simulink model "MMS_ESC_K_B_dither_free"  (R2019b)
settings: Solver=ode4  StartTime=par.sym.TStart  StopTime=par.sym.TStop  FixedStep=par.sym.max_dt  MaxStep=par.sym.max_dt  RelTol=1e-3
undefined symbols (not defined in the file): a1, a1_B, amp, amp_B, b, B_0, B_init, k, K_0, k_B, K_init, k_K, m, N_buff_B, N_buff_K, N_delay, omega, par, R, R_B, T_tran, w_L_B, w_L_K, w_wav
libraries: simulink x2
settings Model: Creator=Vitù  LastModifiedBy=User
settings DataIOCC: SaveFormat=Array  SaveOutput=off  SignalLogging=off  DSMLogging=off  ReturnWorkspaceOutputs=off  TimeSaveName=TIME  OutputSaveName=Yout  OutputOption=SpecifiedOutputTimes  OutputTimes=[par.sym.TStart:par.sym.Outputdt:par.sym.TStop]
settings OptimizationCC: ExpressionDepthLimit=2147483647  LifeSpan=inf
settings DebuggingCC: UnderspecifiedInitializationDetection=Classic  MergeDetectMultiDrivingBlocksExec=none  SolverPrmCheckMsg=warning  AllowSymbolicDim=off  StateNameClashWarn=warning  SFUnexpectedBacktrackingDiag=warning  SFNoUnconditionalDefaultTransitionDiag=warning  SFExecutionAtInitializationDiag=none  ArithmeticOperatorsInVariantConditions=warning
settings HardwareCC: ProdBitPerPointer=32  ProdBitPerSizeT=32  ProdBitPerPtrDiffT=32  ProdLargestAtomicFloat=None  ProdIntDivRoundTo=Undefined  ProdEndianess=Unspecified  ProdWordSize=32  ProdHWDeviceType=32-bit Generic
settings ModelReferenceCC: PropagateSignalLabelsOutOfModel=off
settings SFSimCC: SimUseLocalCustomCode=off  CustomCodeUndefinedFunction=UseInterfaceOnly
settings RTWCC: RTWUseLocalCustomCode=off
settings CodeAppCC: StateflowObjectComments=on
settings GRTTargetCC: TargetLangStandard=C89/C90 (ANSI)  GeneratePreprocessorConditionals=Disable all
settings ConfigComp: CovMetricSettings=dw  CovHtmlReporting=on  CovSaveCumulativeToWorkspaceVar=on  CovSaveSingleToWorkspaceVar=on  CovExternalEMLEnable=off  CovSFcnEnable=off
settings SimscapeCC: SimscapeNormalizeSystem=off
settings ConfigurationSet: Description=SimMechanics 2G

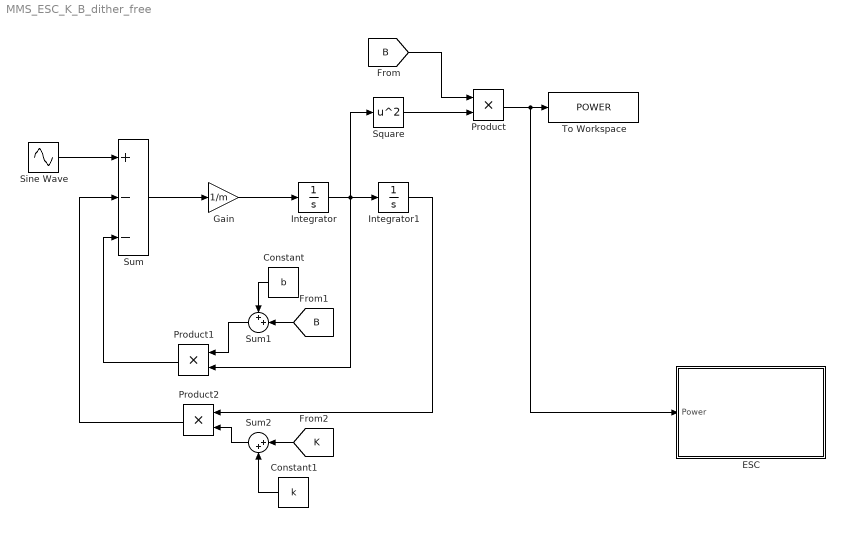
== system MMS_ESC_K_B_dither_free ==
  Constant : Constant  Value=b
  Constant1 : Constant  Value=k
  ESC : Subsystem
  Gain : Gain  Gain=1/m
  Integrator : Integrator
  Integrator1 : Integrator
  Product : Product
  Product1 : Product
  Product2 : Product
  Sine Wave : Sin  Amplitude=par.H  Frequency=w_wav  SampleTime=0
  Square : Math  Operator=square  SignedPower=off  SaturateOnIntegerOverflow=on
  Sum : Sum  Inputs=+--
  Sum1 : Sum  Inputs=++|
  Sum2 : Sum  Inputs=|++
  To Workspace : ToWorkspace  VariableName=POWER  SampleTime=-1
  wires:
  Integrator1/1 -> Product2/1
  Product/1 -> ESC/1(Power), To Workspace/1
  Product1/1 -> Sum/3
  Gain/1 -> Integrator/1
  Square/1 -> Product/2
  Sum/1 -> Gain/1
  Integrator/1 -> Product1/2, Square/1, Integrator1/1
  Product2/1 -> Sum/2
  Sine Wave/1 -> Sum/1
  [B] -> Product/1
  [B] -> Sum1/2
  Sum1/1 -> Product1/1
  Constant/1 -> Sum1/1
  [K] -> Sum2/1
  Sum2/1 -> Product2/2
  Constant1/1 -> Sum2/2

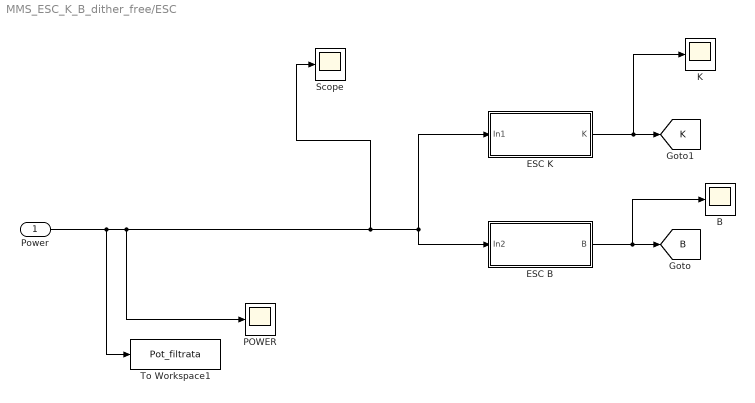
== system MMS_ESC_K_B_dither_free/ESC ==
  Power : Inport
  B : Scope
  ESC B : Subsystem
  ESC K : Subsystem
  K : Scope
  POWER : Scope
  Scope : Scope
  To Workspace1 : ToWorkspace  VariableName=Pot_filtrata  SampleTime=-1
  tag scope: B=global, K=global
  wires:
  Power/1 -> ESC B/1(In2), ESC K/1(In1), Scope/1, POWER/1, To Workspace1/1
  ESC B/1(B) -> B/1, [B]
  ESC K/1(K) -> K/1, [K]

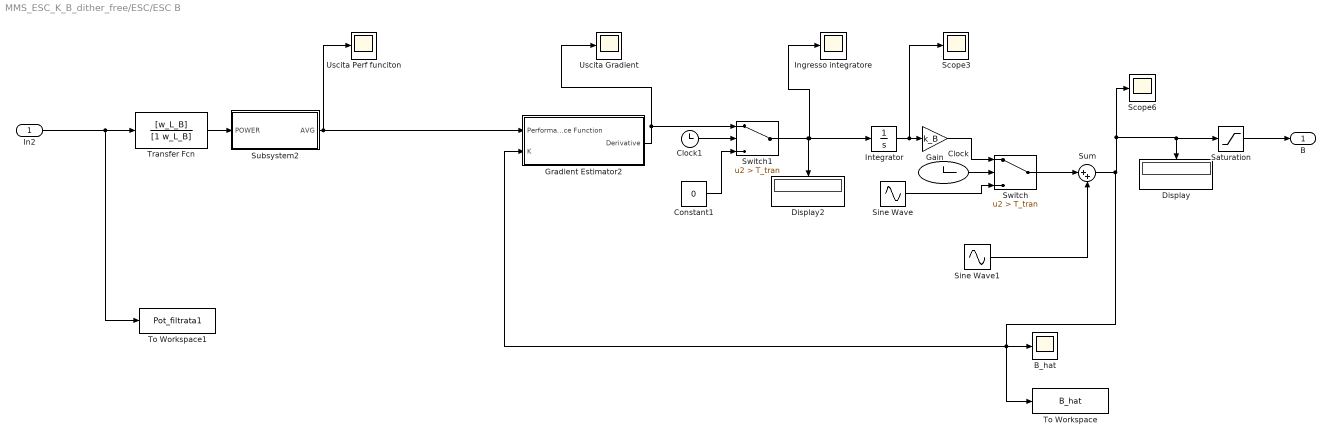
== system MMS_ESC_K_B_dither_free/ESC/ESC B ==
  In2 : Inport
  B_hat : Scope
  Clock : Clock
  Clock1 : Clock
  Constant1 : Constant  Value=0
  Display : Display
  Display2 : Display
  Gain : Gain  Gain=k_B
  Gradient Estimator2 : Subsystem
  Ingresso integratore : Scope
  Integrator : Integrator  InitialCondition=B_init
  Saturation : Saturate  UpperLimit=inf  LowerLimit=-b
  Scope3 : Scope
  Scope6 : Scope
  Sine Wave : Sin  Amplitude=a1_B  Bias=B_0  Frequency=w_wav  SampleTime=0
  Sine Wave1 : Sin  Amplitude=amp_B  Frequency=omega  SampleTime=0
  Subsystem2 : Subsystem
  Sum : Sum  Inputs=|++
  Switch : Switch  Criteria=u2 > Threshold  Threshold=T_tran
  Switch1 : Switch  Criteria=u2 > Threshold  Threshold=T_tran
  To Workspace : ToWorkspace  VariableName=B_hat  SampleTime=-1
  To Workspace1 : ToWorkspace  VariableName=Pot_filtrata1  SampleTime=-1
  Transfer Fcn : TransferFcn  Numerator=[w_L_B]  Denominator=[1 w_L_B]
  Uscita Gradient : Scope
  Uscita Perf funciton : Scope
  B : Outport
  wires:
  Sum/1 -> Saturation/1, Display/1, Scope6/1, Gradient Estimator2/2(K), To Workspace/1, B_hat/1
  Sine Wave/1 -> Switch/3
  Clock/1 -> Switch/2
  Clock1/1 -> Switch1/2
  Switch1/1 -> Integrator/1, Ingresso integratore/1, Display2/1
  Gradient Estimator2/1(Derivative) -> Uscita Gradient/1, Switch1/1
  Switch/1 -> Sum/1
  Constant1/1 -> Switch1/3
  In2/1 -> Transfer Fcn/1, To Workspace1/1
  Sine Wave1/1 -> Sum/2
  Integrator/1 -> Scope3/1, Gain/1
  Gain/1 -> Switch/1
  Transfer Fcn/1 -> Subsystem2/1(POWER)
  Subsystem2/1(AVG) -> Gradient Estimator2/1(Performance Function), Uscita Perf funciton/1
  Saturation/1 -> B/1

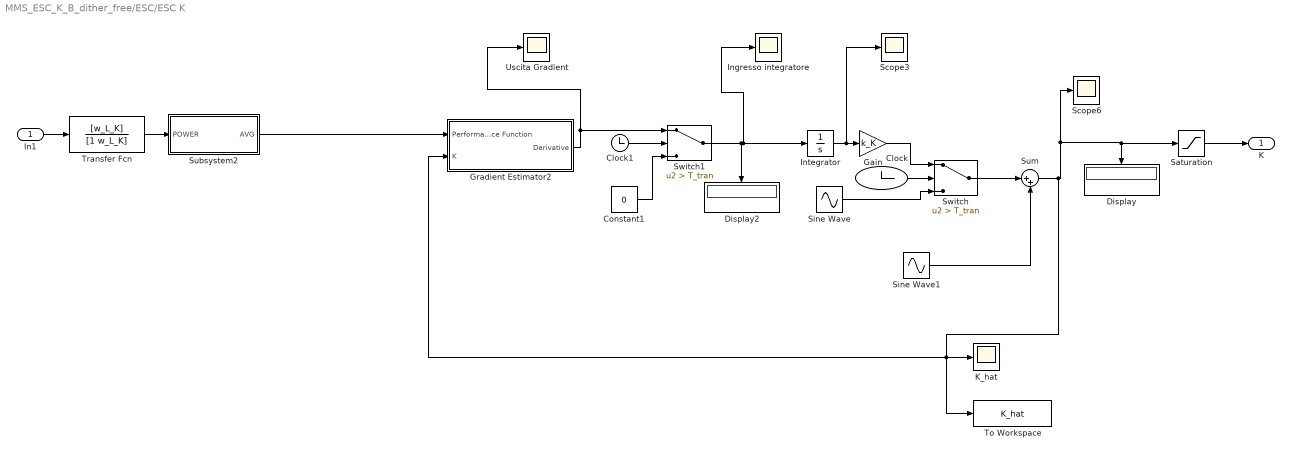
== system MMS_ESC_K_B_dither_free/ESC/ESC K ==
  In1 : Inport
  Clock : Clock
  Clock1 : Clock
  Constant1 : Constant  Value=0
  Display : Display
  Display2 : Display
  Gain : Gain  Gain=k_K
  Gradient Estimator2 : Subsystem
  Ingresso integratore : Scope
  Integrator : Integrator  InitialCondition=K_init
  K_hat : Scope
  Saturation : Saturate  UpperLimit=inf  LowerLimit=-k
  Scope3 : Scope
  Scope6 : Scope
  Sine Wave : Sin  Amplitude=a1  Bias=K_0  Frequency=w_wav  SampleTime=0
  Sine Wave1 : Sin  Amplitude=amp  Frequency=omega  SampleTime=0
  Subsystem2 : Subsystem
  Sum : Sum  Inputs=|++
  Switch : Switch  Criteria=u2 > Threshold  Threshold=T_tran
  Switch1 : Switch  Criteria=u2 > Threshold  Threshold=T_tran
  To Workspace : ToWorkspace  VariableName=K_hat  SampleTime=-1
  Transfer Fcn : TransferFcn  Numerator=[w_L_K]  Denominator=[1 w_L_K]
  Uscita Gradient : Scope
  K : Outport
  wires:
  Gain/1 -> Switch/1
  Switch/1 -> Sum/1
  Sine Wave1/1 -> Sum/2
  In1/1 -> Transfer Fcn/1
  Constant1/1 -> Switch1/3
  Switch1/1 -> Integrator/1, Ingresso integratore/1, Display2/1
  Clock/1 -> Switch/2
  Integrator/1 -> Scope3/1, Gain/1
  Sine Wave/1 -> Switch/3
  Gradient Estimator2/1(Derivative) -> Uscita Gradient/1, Switch1/1
  Sum/1 -> Saturation/1, Display/1, Scope6/1, Gradient Estimator2/2(K), To Workspace/1, K_hat/1
  Clock1/1 -> Switch1/2
  Transfer Fcn/1 -> Subsystem2/1(POWER)
  Subsystem2/1(AVG) -> Gradient Estimator2/1(Performance Function)
  Saturation/1 -> K/1

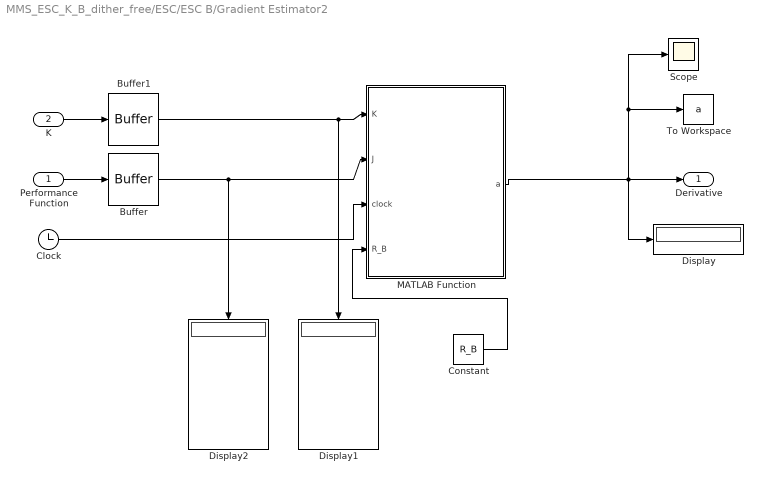
== system MMS_ESC_K_B_dither_free/ESC/ESC B/Gradient Estimator2 ==
  Performance Function : Inport  SampleTime=1
  K : Inport  Port=2  SampleTime=1
  Buffer : Buffer  N=N_buff_B  V=N_buff_B-1  OutputFrames=off
  Buffer1 : Buffer  N=N_buff_B  V=N_buff_B-1  OutputFrames=off
  Clock : Clock
  Constant : Constant  Value=R_B
  Display : Display
  Display1 : Display
  Display2 : Display
  MATLAB Function : MATLAB Function  TreatAsAtomicUnit=on
  Scope : Scope
  To Workspace : ToWorkspace  VariableName=a  SaveFormat=Timeseries  SampleTime=-1
  Derivative : Outport
  wires:
  MATLAB Function/1(a) -> Display/1, Derivative/1, To Workspace/1, Scope/1
  Performance Function/1 -> Buffer/1
  K/1 -> Buffer1/1
  Buffer/1 -> Display2/1, MATLAB Function/2(J)
  Clock/1 -> MATLAB Function/3(clock)
  Buffer1/1 -> MATLAB Function/1(K), Display1/1
  Constant/1 -> MATLAB Function/4(R_B)

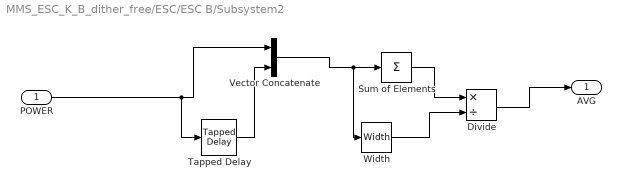
== system MMS_ESC_K_B_dither_free/ESC/ESC B/Subsystem2 ==
  POWER : Inport
  Divide : Product  Inputs=*/
  Sum of Elements : Sum  Inputs=+
  Tapped Delay : simulink/Discrete/Tapped Delay  vinit=0  samptime=-1  NumDelays=N_delay  DelayOrder=Oldest  includeCurrent=off
  Vector Concatenate : Concatenate
  Width : Width
  AVG : Outport
  wires:
  POWER/1 -> Tapped Delay/1, Vector Concatenate/1
  Tapped Delay/1 -> Vector Concatenate/2
  Vector Concatenate/1 -> Width/1, Sum of Elements/1
  Sum of Elements/1 -> Divide/1
  Width/1 -> Divide/2
  Divide/1 -> AVG/1

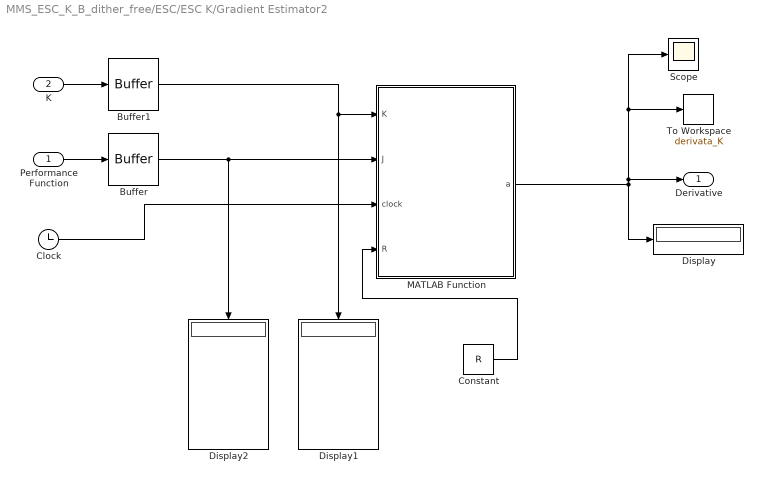
== system MMS_ESC_K_B_dither_free/ESC/ESC K/Gradient Estimator2 ==
  Performance Function : Inport  SampleTime=1
  K : Inport  Port=2  SampleTime=1
  Buffer : Buffer  N=N_buff_K  V=N_buff_K-1  OutputFrames=off
  Buffer1 : Buffer  N=N_buff_K  V=N_buff_K-1  OutputFrames=off
  Clock : Clock
  Constant : Constant  Value=R
  Display : Display
  Display1 : Display
  Display2 : Display
  MATLAB Function : MATLAB Function  TreatAsAtomicUnit=on
  Scope : Scope
  To Workspace : ToWorkspace  VariableName=derivata_K  SampleTime=-1
  Derivative : Outport
  wires:
  MATLAB Function/1(a) -> Derivative/1, To Workspace/1, Scope/1, Display/1
  Performance Function/1 -> Buffer/1
  K/1 -> Buffer1/1
  Buffer/1 -> MATLAB Function/2(J), Display2/1
  Clock/1 -> MATLAB Function/3(clock)
  Buffer1/1 -> MATLAB Function/1(K), Display1/1
  Constant/1 -> MATLAB Function/4(R)

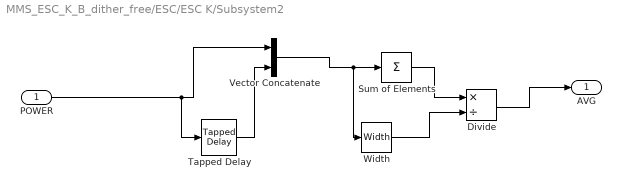
== system MMS_ESC_K_B_dither_free/ESC/ESC K/Subsystem2 ==
  POWER : Inport
  Divide : Product  Inputs=*/
  Sum of Elements : Sum  Inputs=+
  Tapped Delay : simulink/Discrete/Tapped Delay  vinit=0  samptime=-1  NumDelays=N_delay  DelayOrder=Oldest  includeCurrent=off
  Vector Concatenate : Concatenate
  Width : Width
  AVG : Outport
  wires:
  POWER/1 -> Tapped Delay/1, Vector Concatenate/1
  Tapped Delay/1 -> Vector Concatenate/2
  Vector Concatenate/1 -> Width/1, Sum of Elements/1
  Sum of Elements/1 -> Divide/1
  Width/1 -> Divide/2
  Divide/1 -> AVG/1

== matlab function MMS_ESC_K_B_dither_free/ESC/ESC K/Gradient Estimator2/MATLAB Function ==
  data: K input; J input; clock input; a output; R input

function a = LSQ(K,J,clock,R)
if clock > 5
    p = polyfit(K,J,1);
    v = p(1);
%    l = max( [-(log(abs(v))) 9]);
%    l = -log(abs(v));
%     if l<0
%         l=0;
%     end
%   v = v*10^(l);
    s = sign(v);
%    v=abs(v);
%    v = min([v 0.5]);
    a = R*s;
else
    a = 0;
    %l=0;
end

end

== matlab function MMS_ESC_K_B_dither_free/ESC/ESC B/Gradient Estimator2/MATLAB Function ==
  data: K input; J input; clock input; a output; R_B input

function a = LSQ(K,J,clock,R_B)
if clock > 5
    p = polyfit(K,J,1);
    v = p(1);
%    l = max( [-(log(abs(v))) 9]);
%    l = -log(abs(v));
%     if l<0
%         l=0;
%     end
%   v = v*10^(l);
    s = sign(v);
%    v=abs(v);
%    v = min([v 0.5]);
    a = R_B*s;
else
    a = 0;
    %l=0;
end
end
